simulink model "sim4"  (R2022b)
settings: Solver=ode4  StartTime=0  StopTime=60  FixedStep=0.01  RelTol=1e-3
undefined symbols (not defined in the file): Cd_sim, eta_smc, F_grade, K_acceleration, K_Fx_to_Te, K_Te_to_Fx, lambda_smc, p, phi_smc, Rx, Te_max, Te_min, v0
settings Model: Creator=Forough  LastModifiedBy=Forough

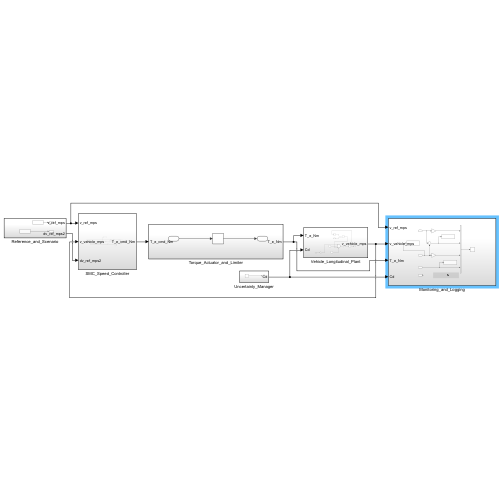
[thumbnail: Simulink's stored preview of the top-level diagram]
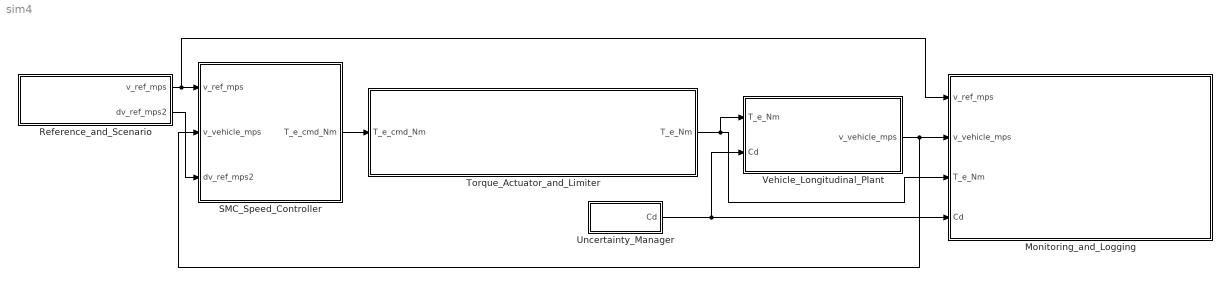
== system sim4 ==
  Monitoring_and_Logging : Subsystem
  Reference_and_Scenario : Subsystem
  SMC_Speed_Controller : Subsystem
  Torque_Actuator_and_Limiter : Subsystem
  Uncertainty_Manager : Subsystem
  Vehicle_Longitudinal_Plant : Subsystem
  wires:
  Uncertainty_Manager/1(Cd) -> Vehicle_Longitudinal_Plant/2(Cd), Monitoring_and_Logging/4(Cd)
  Torque_Actuator_and_Limiter/1(T_e_Nm) -> Monitoring_and_Logging/3(T_e_Nm), Vehicle_Longitudinal_Plant/1(T_e_Nm)
  Vehicle_Longitudinal_Plant/1(v_vehicle_mps) -> SMC_Speed_Controller/2(v_vehicle_mps), Monitoring_and_Logging/2(v_vehicle_mps)
  Reference_and_Scenario/1(v_ref_mps) -> SMC_Speed_Controller/1(v_ref_mps), Monitoring_and_Logging/1(v_ref_mps)
  SMC_Speed_Controller/1(T_e_cmd_Nm) -> Torque_Actuator_and_Limiter/1(T_e_cmd_Nm)
  Reference_and_Scenario/2(dv_ref_mps2) -> SMC_Speed_Controller/3(dv_ref_mps2)

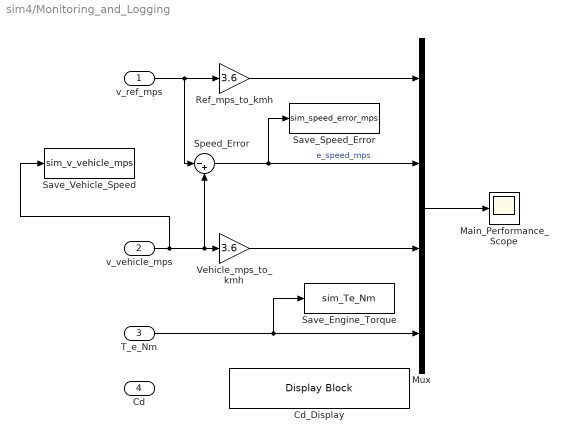
== system sim4/Monitoring_and_Logging ==
  v_ref_mps : Inport
  v_vehicle_mps : Inport  Port=2
  T_e_Nm : Inport  Port=3
  Cd : Inport  Port=4
  Cd_Display : DisplayBlock  LabelPosition=Hide  Transparency=1
  Main_Performance_Scope : Scope
  Mux : Mux
  Ref_mps_to_kmh : Gain  Gain=3.6
  Save_Engine_Torque : ToWorkspace  VariableName=sim_Te_Nm  SampleTime=-1
  Save_Speed_Error : ToWorkspace  VariableName=sim_speed_error_mps  SampleTime=-1
  Save_Vehicle_Speed : ToWorkspace  VariableName=sim_v_vehicle_mps  SampleTime=-1
  Speed_Error : Sum  Inputs=|-+
  Vehicle_mps_to_kmh : Gain  Gain=3.6
  wires:
  v_ref_mps/1 -> Speed_Error/1, Ref_mps_to_kmh/1
  Ref_mps_to_kmh/1 -> Mux/1
  v_vehicle_mps/1 -> Save_Vehicle_Speed/1, Speed_Error/2, Vehicle_mps_to_kmh/1
  Vehicle_mps_to_kmh/1 -> Mux/3
  Speed_Error/1 -> Save_Speed_Error/1, Mux/2  "e_speed_mps"
  T_e_Nm/1 -> Save_Engine_Torque/1, Mux/4
  Mux/1 -> Main_Performance_Scope/1

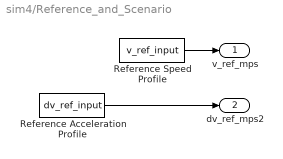
== system sim4/Reference_and_Scenario ==
  Reference Acceleration Profile : FromWorkspace  VariableName=dv_ref_input
  Reference Speed Profile : FromWorkspace  VariableName=v_ref_input
  v_ref_mps : Outport
  dv_ref_mps2 : Outport  Port=2
  wires:
  Reference Speed Profile/1 -> v_ref_mps/1
  Reference Acceleration Profile/1 -> dv_ref_mps2/1

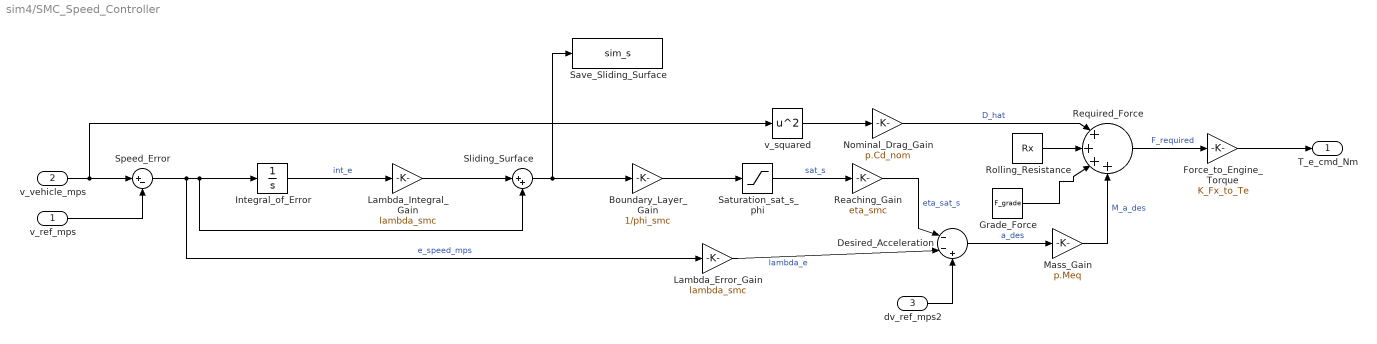
== system sim4/SMC_Speed_Controller ==
  v_ref_mps : Inport
  v_vehicle_mps : Inport  Port=2
  dv_ref_mps2 : Inport  Port=3
  Boundary_Layer_Gain : Gain  Gain=1/phi_smc
  Desired_Acceleration : Sum  Inputs=|--+
  Force_to_Engine_Torque : Gain  Gain=K_Fx_to_Te
  Grade_Force : Constant  Value=F_grade
  Integral_of_Error : Integrator
  Lambda_Error_Gain : Gain  Gain=lambda_smc
  Lambda_Integral_Gain : Gain  Gain=lambda_smc
  Mass_Gain : Gain  Gain=p.Meq
  Nominal_Drag_Gain : Gain  Gain=p.Cd_nom
  Reaching_Gain : Gain  Gain=eta_smc
  Required_Force : Sum  Inputs=|++++
  Rolling_Resistance : Constant  Value=Rx
  Saturation_sat_s_phi : Saturate  UpperLimit=1  LowerLimit=-1
  Save_Sliding_Surface : ToWorkspace  VariableName=sim_s  SampleTime=-1
  Sliding_Surface : Sum  Inputs=|++
  Speed_Error : Sum  Inputs=|+-
  v_squared : Math  Operator=square
  T_e_cmd_Nm : Outport
  wires:
  Force_to_Engine_Torque/1 -> T_e_cmd_Nm/1
  v_vehicle_mps/1 -> v_squared/1, Speed_Error/1
  v_ref_mps/1 -> Speed_Error/2
  Speed_Error/1 -> Lambda_Error_Gain/1, Sliding_Surface/2, Integral_of_Error/1  "e_speed_mps"
  Integral_of_Error/1 -> Lambda_Integral_Gain/1  "int_e"
  Lambda_Integral_Gain/1 -> Sliding_Surface/1
  Sliding_Surface/1 -> Boundary_Layer_Gain/1, Save_Sliding_Surface/1
  Boundary_Layer_Gain/1 -> Saturation_sat_s_phi/1
  Saturation_sat_s_phi/1 -> Reaching_Gain/1  "sat_s"
  Lambda_Error_Gain/1 -> Desired_Acceleration/2  "lambda_e"
  Reaching_Gain/1 -> Desired_Acceleration/1  "eta_sat_s"
  dv_ref_mps2/1 -> Desired_Acceleration/3
  Desired_Acceleration/1 -> Mass_Gain/1  "a_des"
  Mass_Gain/1 -> Required_Force/4  "M_a_des"
  v_squared/1 -> Nominal_Drag_Gain/1
  Nominal_Drag_Gain/1 -> Required_Force/1  "D_hat"
  Rolling_Resistance/1 -> Required_Force/2
  Grade_Force/1 -> Required_Force/3
  Required_Force/1 -> Force_to_Engine_Torque/1  "F_required"

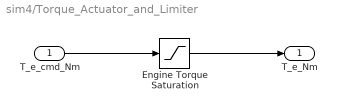
== system sim4/Torque_Actuator_and_Limiter ==
  T_e_cmd_Nm : Inport
  Engine Torque Saturation : Saturate  UpperLimit=Te_max  LowerLimit=Te_min
  T_e_Nm : Outport
  wires:
  T_e_cmd_Nm/1 -> Engine Torque Saturation/1
  Engine Torque Saturation/1 -> T_e_Nm/1

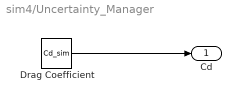
== system sim4/Uncertainty_Manager ==
  Drag Coefficient : Constant  Value=Cd_sim
  Cd : Outport
  wires:
  Drag Coefficient/1 -> Cd/1

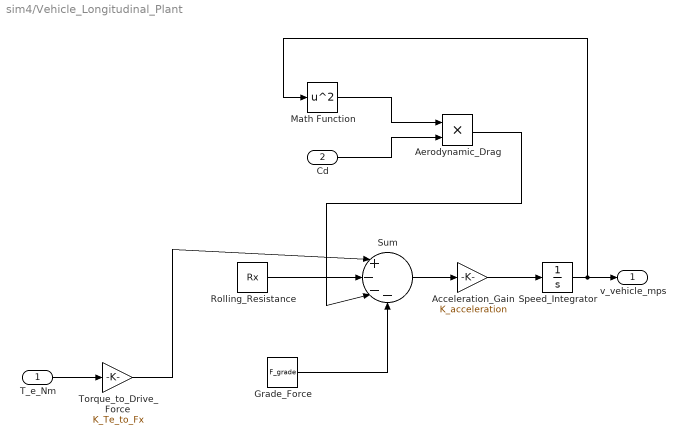
== system sim4/Vehicle_Longitudinal_Plant ==
  T_e_Nm : Inport
  Cd : Inport  Port=2
  Acceleration_Gain : Gain  Gain=K_acceleration
  Aerodynamic_Drag : Product
  Grade_Force : Constant  Value=F_grade
  Math Function : Math  Operator=square
  Rolling_Resistance : Constant  Value=Rx
  Speed_Integrator : Integrator  InitialCondition=v0
  Sum : Sum  Inputs=|+---
  Torque_to_Drive_Force : Gain  Gain=K_Te_to_Fx
  v_vehicle_mps : Outport
  wires:
  Cd/1 -> Aerodynamic_Drag/2
  T_e_Nm/1 -> Torque_to_Drive_Force/1
  Torque_to_Drive_Force/1 -> Sum/1
  Rolling_Resistance/1 -> Sum/2
  Acceleration_Gain/1 -> Speed_Integrator/1
  Sum/1 -> Acceleration_Gain/1
  Speed_Integrator/1 -> Math Function/1, v_vehicle_mps/1
  Grade_Force/1 -> Sum/4
  Math Function/1 -> Aerodynamic_Drag/1
  Aerodynamic_Drag/1 -> Sum/3
